simulink model "TST_EISGov_SelectTrqLim"  (R2016b)
settings: Solver=FixedStepDiscrete  StartTime=0.0  StopTime=simTime  FixedStep=sampleTime  RelTol=1e-3
values from neighbouring files (symbols this model uses):
  testCase = 1    [initTST_EISGov_SelectTrqLim_001.m]    (also in initTST_EISGov_SelectTrqLim_002.m = 2; initTST_EISGov_SelectTrqLim_003.m = 3)
libraries: simulink x19, UnitTest_Lib x15
settings Model: Creator=zhengjinyan  LastModifiedBy=zhengjinyan
settings DebuggingCC: SignalRangeChecking=error

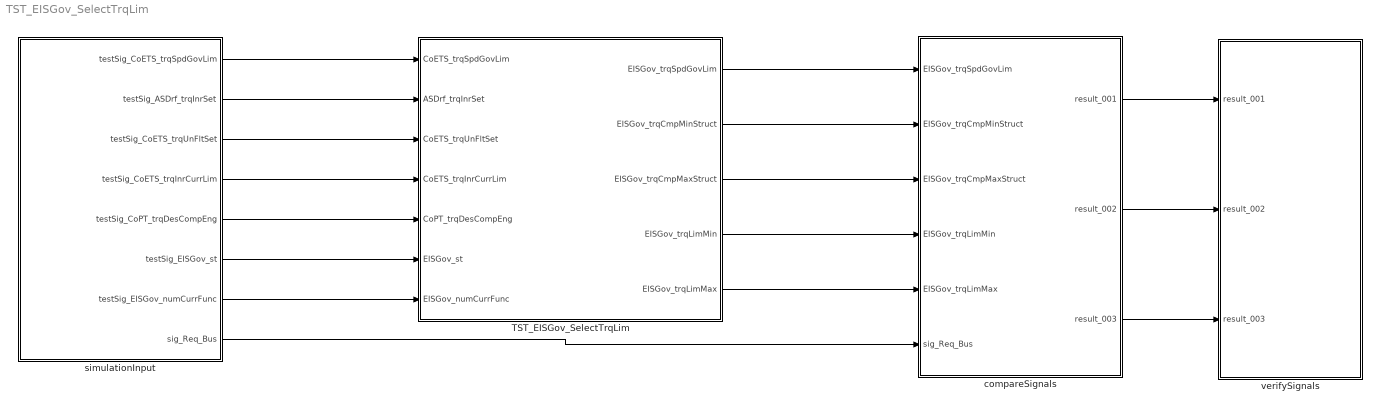
== system TST_EISGov_SelectTrqLim ==
  TST_EISGov_SelectTrqLim : Subsystem
  compareSignals : Subsystem
  simulationInput : Subsystem
  verifySignals : Subsystem
  wires:
  simulationInput/1(testSig_CoETS_trqSpdGovLim) -> TST_EISGov_SelectTrqLim/1(CoETS_trqSpdGovLim)
  simulationInput/2(testSig_ASDrf_trqInrSet) -> TST_EISGov_SelectTrqLim/2(ASDrf_trqInrSet)
  simulationInput/3(testSig_CoETS_trqUnFltSet) -> TST_EISGov_SelectTrqLim/3(CoETS_trqUnFltSet)
  simulationInput/4(testSig_CoETS_trqInrCurrLim) -> TST_EISGov_SelectTrqLim/4(CoETS_trqInrCurrLim)
  simulationInput/5(testSig_CoPT_trqDesCompEng) -> TST_EISGov_SelectTrqLim/5(CoPT_trqDesCompEng)
  simulationInput/6(testSig_EISGov_st) -> TST_EISGov_SelectTrqLim/6(EISGov_st)
  simulationInput/7(testSig_EISGov_numCurrFunc) -> TST_EISGov_SelectTrqLim/7(EISGov_numCurrFunc)
  TST_EISGov_SelectTrqLim/1(EISGov_trqSpdGovLim) -> compareSignals/1(EISGov_trqSpdGovLim)
  TST_EISGov_SelectTrqLim/2(EISGov_trqCmpMinStruct) -> compareSignals/2(EISGov_trqCmpMinStruct)
  TST_EISGov_SelectTrqLim/3(EISGov_trqCmpMaxStruct) -> compareSignals/3(EISGov_trqCmpMaxStruct)
  TST_EISGov_SelectTrqLim/4(EISGov_trqLimMin) -> compareSignals/4(EISGov_trqLimMin)
  TST_EISGov_SelectTrqLim/5(EISGov_trqLimMax) -> compareSignals/5(EISGov_trqLimMax)
  simulationInput/8(sig_Req_Bus) -> compareSignals/6(sig_Req_Bus)
  compareSignals/1(result_001) -> verifySignals/1(result_001)
  compareSignals/2(result_002) -> verifySignals/2(result_002)
  compareSignals/3(result_003) -> verifySignals/3(result_003)

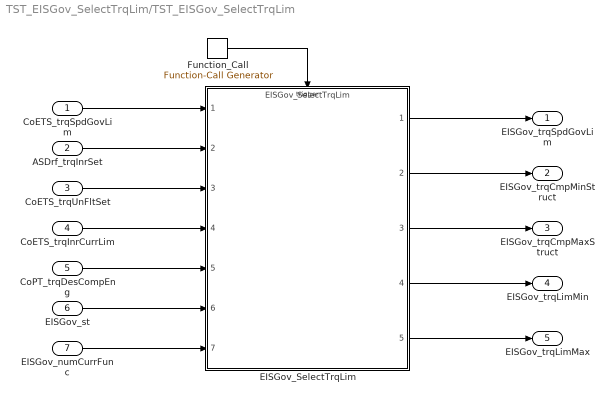
== system TST_EISGov_SelectTrqLim/TST_EISGov_SelectTrqLim ==
  CoETS_trqSpdGovLim : Inport
  ASDrf_trqInrSet : Inport  Port=2
  CoETS_trqUnFltSet : Inport  Port=3
  CoETS_trqInrCurrLim : Inport  Port=4
  CoPT_trqDesCompEng : Inport  Port=5
  EISGov_st : Inport  Port=6
  EISGov_numCurrFunc : Inport  Port=7
  EISGov_SelectTrqLim : ModelReference  ModelNameDialog=EISGov_SelectTrqLim  SimulationMode=Normal  ModelReferenceVersion=1.26  TriggerPortName=function  TriggerPortTriggerType=function-call  TriggerPortStatesWhenEnabling=held
  Function_Call : simulink/Ports & Subsystems/Function-Call Generator  sample_time=sampleTime  numberOfIterations=1
  EISGov_trqSpdGovLim : Outport
  EISGov_trqCmpMinStruct : Outport  Port=2
  EISGov_trqCmpMaxStruct : Outport  Port=3
  EISGov_trqLimMin : Outport  Port=4
  EISGov_trqLimMax : Outport  Port=5
  wires:
  Function_Call/1 -> EISGov_SelectTrqLim/Trigger
  CoETS_trqSpdGovLim/1 -> EISGov_SelectTrqLim/1
  ASDrf_trqInrSet/1 -> EISGov_SelectTrqLim/2
  CoETS_trqUnFltSet/1 -> EISGov_SelectTrqLim/3
  CoETS_trqInrCurrLim/1 -> EISGov_SelectTrqLim/4
  CoPT_trqDesCompEng/1 -> EISGov_SelectTrqLim/5
  EISGov_st/1 -> EISGov_SelectTrqLim/6
  EISGov_numCurrFunc/1 -> EISGov_SelectTrqLim/7
  EISGov_SelectTrqLim/1 -> EISGov_trqSpdGovLim/1
  EISGov_SelectTrqLim/2 -> EISGov_trqCmpMinStruct/1
  EISGov_SelectTrqLim/3 -> EISGov_trqCmpMaxStruct/1
  EISGov_SelectTrqLim/4 -> EISGov_trqLimMin/1
  EISGov_SelectTrqLim/5 -> EISGov_trqLimMax/1

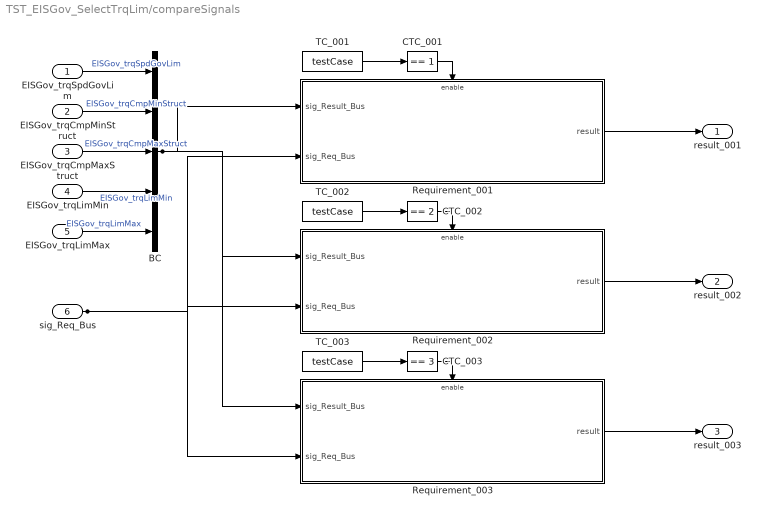
== system TST_EISGov_SelectTrqLim/compareSignals ==
  EISGov_trqSpdGovLim : Inport
  EISGov_trqCmpMinStruct : Inport  Port=2
  EISGov_trqCmpMaxStruct : Inport  Port=3
  EISGov_trqLimMin : Inport  Port=4
  EISGov_trqLimMax : Inport  Port=5
  sig_Req_Bus : Inport  Port=6
  BC : BusCreator  Inputs=5
  CTC_001 : simulink/Logic and Bit Operations/Compare To Constant  relop===  const=1  OutDataTypeStr=boolean
  CTC_002 : simulink/Logic and Bit Operations/Compare To Constant  relop===  const=2  OutDataTypeStr=boolean
  CTC_003 : simulink/Logic and Bit Operations/Compare To Constant  relop===  const=3  OutDataTypeStr=boolean
  Requirement_001 : Subsystem
  Requirement_002 : Subsystem
  Requirement_003 : Subsystem
  TC_001 : Constant  Value=testCase
  TC_002 : Constant  Value=testCase
  TC_003 : Constant  Value=testCase
  result_001 : Outport
  result_002 : Outport  Port=2
  result_003 : Outport  Port=3
  wires:
  EISGov_trqSpdGovLim/1 -> BC/1  "EISGov_trqSpdGovLim"
  EISGov_trqCmpMinStruct/1 -> BC/2  "EISGov_trqCmpMinStruct"
  EISGov_trqCmpMaxStruct/1 -> BC/3  "EISGov_trqCmpMaxStruct"
  EISGov_trqLimMin/1 -> BC/4  "EISGov_trqLimMin"
  EISGov_trqLimMax/1 -> BC/5  "EISGov_trqLimMax"
  TC_001/1 -> CTC_001/1
  CTC_001/1 -> Requirement_001/Enable
  sig_Req_Bus/1 -> Requirement_001/2(sig_Req_Bus), Requirement_002/2(sig_Req_Bus), Requirement_003/2(sig_Req_Bus)
  BC/1 -> Requirement_001/1(sig_Result_Bus), Requirement_002/1(sig_Result_Bus), Requirement_003/1(sig_Result_Bus)
  Requirement_001/1(result) -> result_001/1
  TC_002/1 -> CTC_002/1
  CTC_002/1 -> Requirement_002/Enable
  Requirement_002/1(result) -> result_002/1
  TC_003/1 -> CTC_003/1
  CTC_003/1 -> Requirement_003/Enable
  Requirement_003/1(result) -> result_003/1

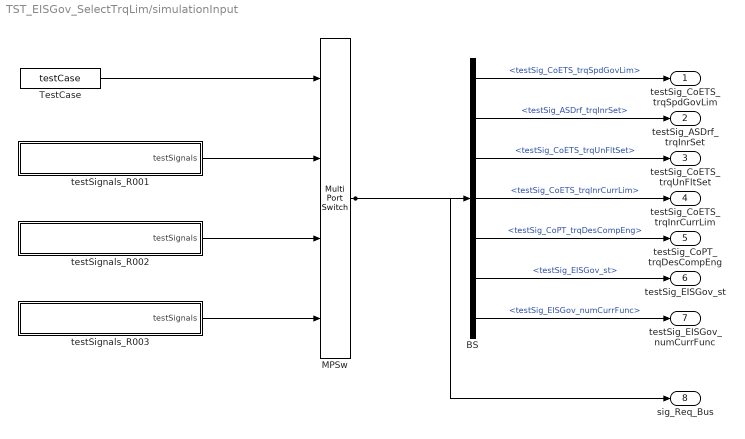
== system TST_EISGov_SelectTrqLim/simulationInput ==
  BS : BusSelector  OutputSignals=testSig_CoETS_trqSpdGovLim,testSig_ASDrf_trqInrSet,testSig_CoETS_trqUnFltSet,testSig_CoETS_trqInrCurrLim,testSig_CoPT_trqDesCompEng,testSig_EISGov_st,testSig_EISGov_numCurrFunc
  MPSw : MultiPortSwitch  SaturateOnIntegerOverflow=on  InputSameDT=on
  TestCase : Constant  Value=testCase
  testSignals_R001 : Subsystem
  testSignals_R002 : Subsystem
  testSignals_R003 : Subsystem
  testSig_CoETS_trqSpdGovLim : Outport
  testSig_ASDrf_trqInrSet : Outport  Port=2
  testSig_CoETS_trqUnFltSet : Outport  Port=3
  testSig_CoETS_trqInrCurrLim : Outport  Port=4
  testSig_CoPT_trqDesCompEng : Outport  Port=5
  testSig_EISGov_st : Outport  Port=6
  testSig_EISGov_numCurrFunc : Outport  Port=7
  sig_Req_Bus : Outport  Port=8
  wires:
  BS/1 -> testSig_CoETS_trqSpdGovLim/1  "<testSig_CoETS_trqSpdGovLim>"
  BS/2 -> testSig_ASDrf_trqInrSet/1  "<testSig_ASDrf_trqInrSet>"
  BS/3 -> testSig_CoETS_trqUnFltSet/1  "<testSig_CoETS_trqUnFltSet>"
  BS/4 -> testSig_CoETS_trqInrCurrLim/1  "<testSig_CoETS_trqInrCurrLim>"
  BS/5 -> testSig_CoPT_trqDesCompEng/1  "<testSig_CoPT_trqDesCompEng>"
  BS/6 -> testSig_EISGov_st/1  "<testSig_EISGov_st>"
  BS/7 -> testSig_EISGov_numCurrFunc/1  "<testSig_EISGov_numCurrFunc>"
  MPSw/1 -> BS/1, sig_Req_Bus/1
  TestCase/1 -> MPSw/1
  testSignals_R001/1(testSignals) -> MPSw/2
  testSignals_R002/1(testSignals) -> MPSw/3
  testSignals_R003/1(testSignals) -> MPSw/4

== system TST_EISGov_SelectTrqLim/verifySignals ==
  result_001 : Inport
  result_002 : Inport  Port=2
  result_003 : Inport  Port=3
  Assertion_001 : Assertion  Enabled=off
  Assertion_002 : Assertion  Enabled=off
  Assertion_003 : Assertion  Enabled=off
  wires:
  result_001/1 -> Assertion_001/1
  result_002/1 -> Assertion_002/1
  result_003/1 -> Assertion_003/1

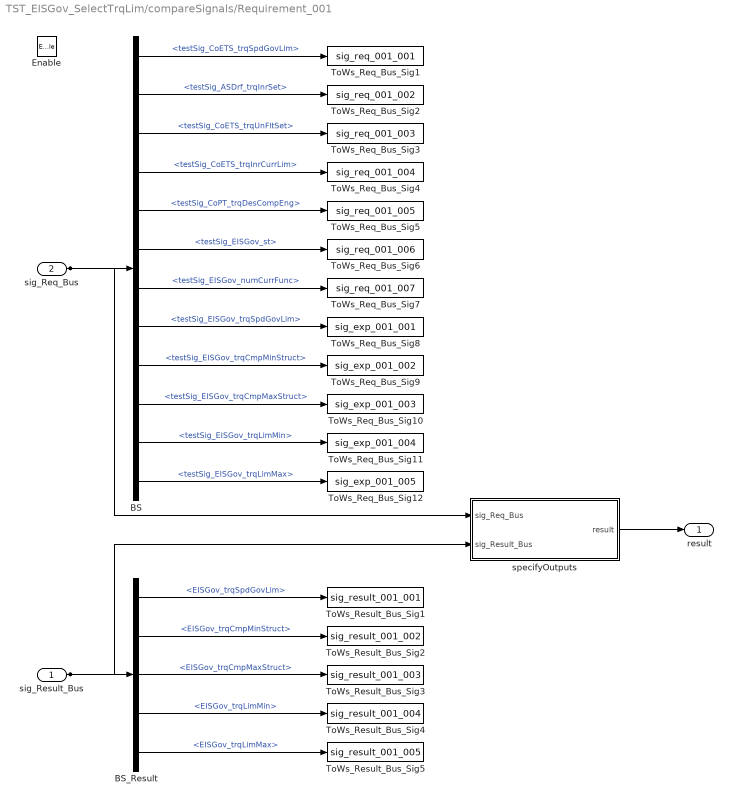
== system TST_EISGov_SelectTrqLim/compareSignals/Requirement_001 ==
  sig_Result_Bus : Inport
  sig_Req_Bus : Inport  Port=2
  Enable : EnablePort
  BS : BusSelector  OutputSignals=testSig_CoETS_trqSpdGovLim,testSig_ASDrf_trqInrSet,testSig_CoETS_trqUnFltSet,testSig_CoETS_trqInrCurrLim,testSig_CoPT_trqDesCompEng,testSig_EISGov_st,testSig_EISGov_numCurrFunc,testSig_EISGov_trqSpdGovLim,testSig_EISGov_trqCmpMinStruct,testSig_EISGov_trqCmpMaxStruct,testSig_EISGov_trqLimMin,testSig_EISGov_trqLimMax
  BS_Result : BusSelector  OutputSignals=EISGov_trqSpdGovLim,EISGov_trqCmpMinStruct,EISGov_trqCmpMaxStruct,EISGov_trqLimMin,EISGov_trqLimMax
  ToWs_Req_Bus_Sig1 : ToWorkspace  VariableName=sig_req_001_001  SaveFormat=Structure With Time
  ToWs_Req_Bus_Sig10 : ToWorkspace  VariableName=sig_exp_001_003  SaveFormat=Structure With Time
  ToWs_Req_Bus_Sig11 : ToWorkspace  VariableName=sig_exp_001_004  SaveFormat=Structure With Time
  ToWs_Req_Bus_Sig12 : ToWorkspace  VariableName=sig_exp_001_005  SaveFormat=Structure With Time
  ToWs_Req_Bus_Sig2 : ToWorkspace  VariableName=sig_req_001_002  SaveFormat=Structure With Time
  ToWs_Req_Bus_Sig3 : ToWorkspace  VariableName=sig_req_001_003  SaveFormat=Structure With Time
  ToWs_Req_Bus_Sig4 : ToWorkspace  VariableName=sig_req_001_004  SaveFormat=Structure With Time
  ToWs_Req_Bus_Sig5 : ToWorkspace  VariableName=sig_req_001_005  SaveFormat=Structure With Time
  ToWs_Req_Bus_Sig6 : ToWorkspace  VariableName=sig_req_001_006  SaveFormat=Structure With Time
  ToWs_Req_Bus_Sig7 : ToWorkspace  VariableName=sig_req_001_007  SaveFormat=Structure With Time
  ToWs_Req_Bus_Sig8 : ToWorkspace  VariableName=sig_exp_001_001  SaveFormat=Structure With Time
  ToWs_Req_Bus_Sig9 : ToWorkspace  VariableName=sig_exp_001_002  SaveFormat=Structure With Time
  ToWs_Result_Bus_Sig1 : ToWorkspace  VariableName=sig_result_001_001  SaveFormat=Structure With Time
  ToWs_Result_Bus_Sig2 : ToWorkspace  VariableName=sig_result_001_002  SaveFormat=Structure With Time
  ToWs_Result_Bus_Sig3 : ToWorkspace  VariableName=sig_result_001_003  SaveFormat=Structure With Time
  ToWs_Result_Bus_Sig4 : ToWorkspace  VariableName=sig_result_001_004  SaveFormat=Structure With Time
  ToWs_Result_Bus_Sig5 : ToWorkspace  VariableName=sig_result_001_005  SaveFormat=Structure With Time
  specifyOutputs : Subsystem
  result : Outport
  wires:
  sig_Req_Bus/1 -> BS/1, specifyOutputs/1(sig_Req_Bus)
  BS/1 -> ToWs_Req_Bus_Sig1/1  "<testSig_CoETS_trqSpdGovLim>"
  BS/2 -> ToWs_Req_Bus_Sig2/1  "<testSig_ASDrf_trqInrSet>"
  BS/3 -> ToWs_Req_Bus_Sig3/1  "<testSig_CoETS_trqUnFltSet>"
  BS/4 -> ToWs_Req_Bus_Sig4/1  "<testSig_CoETS_trqInrCurrLim>"
  BS/5 -> ToWs_Req_Bus_Sig5/1  "<testSig_CoPT_trqDesCompEng>"
  BS/6 -> ToWs_Req_Bus_Sig6/1  "<testSig_EISGov_st>"
  BS/7 -> ToWs_Req_Bus_Sig7/1  "<testSig_EISGov_numCurrFunc>"
  BS/8 -> ToWs_Req_Bus_Sig8/1  "<testSig_EISGov_trqSpdGovLim>"
  BS/9 -> ToWs_Req_Bus_Sig9/1  "<testSig_EISGov_trqCmpMinStruct>"
  BS/10 -> ToWs_Req_Bus_Sig10/1  "<testSig_EISGov_trqCmpMaxStruct>"
  BS/11 -> ToWs_Req_Bus_Sig11/1  "<testSig_EISGov_trqLimMin>"
  BS/12 -> ToWs_Req_Bus_Sig12/1  "<testSig_EISGov_trqLimMax>"
  sig_Result_Bus/1 -> BS_Result/1, specifyOutputs/2(sig_Result_Bus)
  BS_Result/1 -> ToWs_Result_Bus_Sig1/1  "<EISGov_trqSpdGovLim>"
  BS_Result/2 -> ToWs_Result_Bus_Sig2/1  "<EISGov_trqCmpMinStruct>"
  BS_Result/3 -> ToWs_Result_Bus_Sig3/1  "<EISGov_trqCmpMaxStruct>"
  BS_Result/4 -> ToWs_Result_Bus_Sig4/1  "<EISGov_trqLimMin>"
  BS_Result/5 -> ToWs_Result_Bus_Sig5/1  "<EISGov_trqLimMax>"
  specifyOutputs/1(result) -> result/1

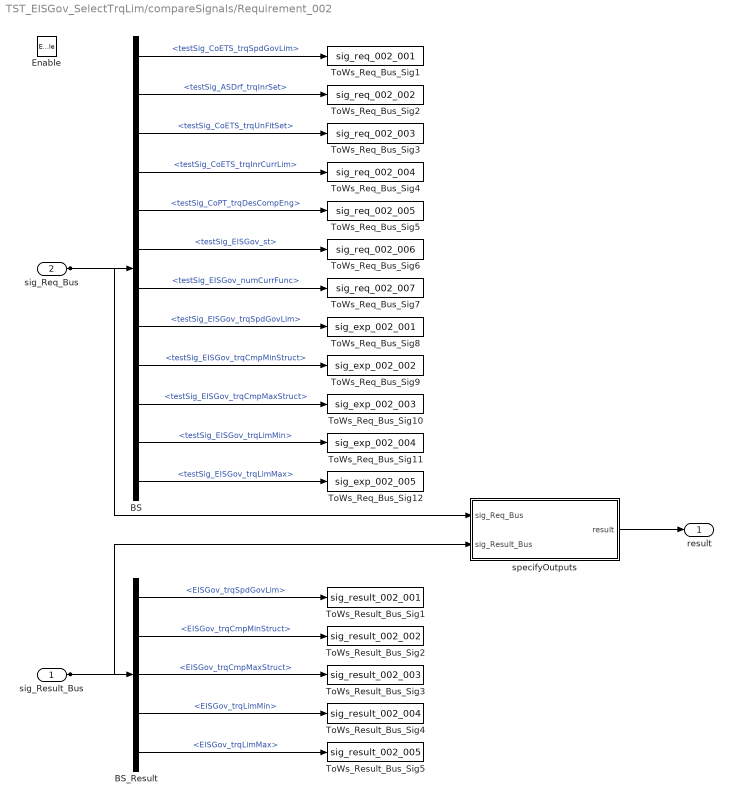
== system TST_EISGov_SelectTrqLim/compareSignals/Requirement_002 ==
  sig_Result_Bus : Inport
  sig_Req_Bus : Inport  Port=2
  Enable : EnablePort
  BS : BusSelector  OutputSignals=testSig_CoETS_trqSpdGovLim,testSig_ASDrf_trqInrSet,testSig_CoETS_trqUnFltSet,testSig_CoETS_trqInrCurrLim,testSig_CoPT_trqDesCompEng,testSig_EISGov_st,testSig_EISGov_numCurrFunc,testSig_EISGov_trqSpdGovLim,testSig_EISGov_trqCmpMinStruct,testSig_EISGov_trqCmpMaxStruct,testSig_EISGov_trqLimMin,testSig_EISGov_trqLimMax
  BS_Result : BusSelector  OutputSignals=EISGov_trqSpdGovLim,EISGov_trqCmpMinStruct,EISGov_trqCmpMaxStruct,EISGov_trqLimMin,EISGov_trqLimMax
  ToWs_Req_Bus_Sig1 : ToWorkspace  VariableName=sig_req_002_001  SaveFormat=Structure With Time
  ToWs_Req_Bus_Sig10 : ToWorkspace  VariableName=sig_exp_002_003  SaveFormat=Structure With Time
  ToWs_Req_Bus_Sig11 : ToWorkspace  VariableName=sig_exp_002_004  SaveFormat=Structure With Time
  ToWs_Req_Bus_Sig12 : ToWorkspace  VariableName=sig_exp_002_005  SaveFormat=Structure With Time
  ToWs_Req_Bus_Sig2 : ToWorkspace  VariableName=sig_req_002_002  SaveFormat=Structure With Time
  ToWs_Req_Bus_Sig3 : ToWorkspace  VariableName=sig_req_002_003  SaveFormat=Structure With Time
  ToWs_Req_Bus_Sig4 : ToWorkspace  VariableName=sig_req_002_004  SaveFormat=Structure With Time
  ToWs_Req_Bus_Sig5 : ToWorkspace  VariableName=sig_req_002_005  SaveFormat=Structure With Time
  ToWs_Req_Bus_Sig6 : ToWorkspace  VariableName=sig_req_002_006  SaveFormat=Structure With Time
  ToWs_Req_Bus_Sig7 : ToWorkspace  VariableName=sig_req_002_007  SaveFormat=Structure With Time
  ToWs_Req_Bus_Sig8 : ToWorkspace  VariableName=sig_exp_002_001  SaveFormat=Structure With Time
  ToWs_Req_Bus_Sig9 : ToWorkspace  VariableName=sig_exp_002_002  SaveFormat=Structure With Time
  ToWs_Result_Bus_Sig1 : ToWorkspace  VariableName=sig_result_002_001  SaveFormat=Structure With Time
  ToWs_Result_Bus_Sig2 : ToWorkspace  VariableName=sig_result_002_002  SaveFormat=Structure With Time
  ToWs_Result_Bus_Sig3 : ToWorkspace  VariableName=sig_result_002_003  SaveFormat=Structure With Time
  ToWs_Result_Bus_Sig4 : ToWorkspace  VariableName=sig_result_002_004  SaveFormat=Structure With Time
  ToWs_Result_Bus_Sig5 : ToWorkspace  VariableName=sig_result_002_005  SaveFormat=Structure With Time
  specifyOutputs : Subsystem
  result : Outport
  wires:
  sig_Req_Bus/1 -> BS/1, specifyOutputs/1(sig_Req_Bus)
  BS/1 -> ToWs_Req_Bus_Sig1/1  "<testSig_CoETS_trqSpdGovLim>"
  BS/2 -> ToWs_Req_Bus_Sig2/1  "<testSig_ASDrf_trqInrSet>"
  BS/3 -> ToWs_Req_Bus_Sig3/1  "<testSig_CoETS_trqUnFltSet>"
  BS/4 -> ToWs_Req_Bus_Sig4/1  "<testSig_CoETS_trqInrCurrLim>"
  BS/5 -> ToWs_Req_Bus_Sig5/1  "<testSig_CoPT_trqDesCompEng>"
  BS/6 -> ToWs_Req_Bus_Sig6/1  "<testSig_EISGov_st>"
  BS/7 -> ToWs_Req_Bus_Sig7/1  "<testSig_EISGov_numCurrFunc>"
  BS/8 -> ToWs_Req_Bus_Sig8/1  "<testSig_EISGov_trqSpdGovLim>"
  BS/9 -> ToWs_Req_Bus_Sig9/1  "<testSig_EISGov_trqCmpMinStruct>"
  BS/10 -> ToWs_Req_Bus_Sig10/1  "<testSig_EISGov_trqCmpMaxStruct>"
  BS/11 -> ToWs_Req_Bus_Sig11/1  "<testSig_EISGov_trqLimMin>"
  BS/12 -> ToWs_Req_Bus_Sig12/1  "<testSig_EISGov_trqLimMax>"
  sig_Result_Bus/1 -> BS_Result/1, specifyOutputs/2(sig_Result_Bus)
  BS_Result/1 -> ToWs_Result_Bus_Sig1/1  "<EISGov_trqSpdGovLim>"
  BS_Result/2 -> ToWs_Result_Bus_Sig2/1  "<EISGov_trqCmpMinStruct>"
  BS_Result/3 -> ToWs_Result_Bus_Sig3/1  "<EISGov_trqCmpMaxStruct>"
  BS_Result/4 -> ToWs_Result_Bus_Sig4/1  "<EISGov_trqLimMin>"
  BS_Result/5 -> ToWs_Result_Bus_Sig5/1  "<EISGov_trqLimMax>"
  specifyOutputs/1(result) -> result/1

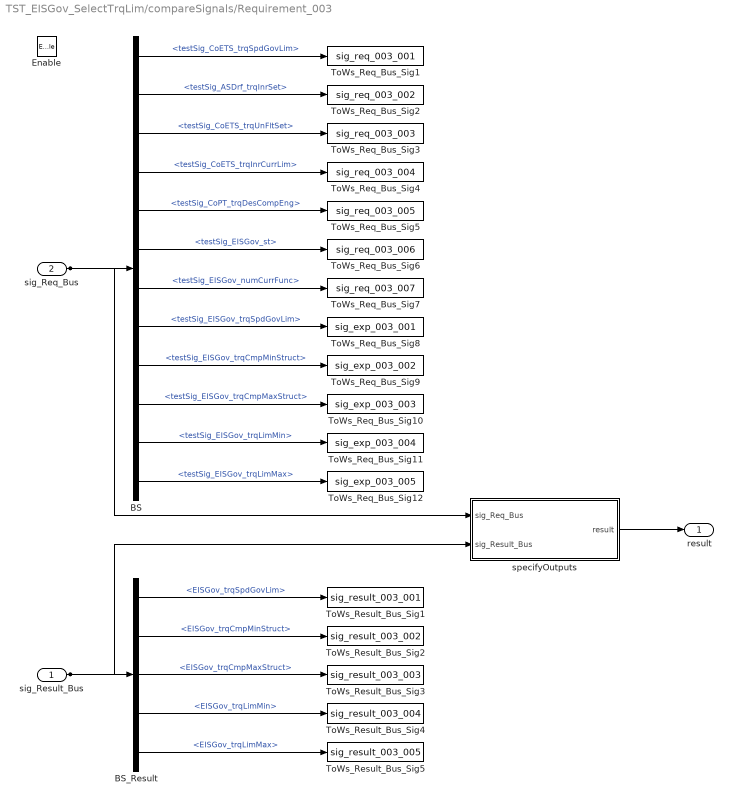
== system TST_EISGov_SelectTrqLim/compareSignals/Requirement_003 ==
  sig_Result_Bus : Inport
  sig_Req_Bus : Inport  Port=2
  Enable : EnablePort
  BS : BusSelector  OutputSignals=testSig_CoETS_trqSpdGovLim,testSig_ASDrf_trqInrSet,testSig_CoETS_trqUnFltSet,testSig_CoETS_trqInrCurrLim,testSig_CoPT_trqDesCompEng,testSig_EISGov_st,testSig_EISGov_numCurrFunc,testSig_EISGov_trqSpdGovLim,testSig_EISGov_trqCmpMinStruct,testSig_EISGov_trqCmpMaxStruct,testSig_EISGov_trqLimMin,testSig_EISGov_trqLimMax
  BS_Result : BusSelector  OutputSignals=EISGov_trqSpdGovLim,EISGov_trqCmpMinStruct,EISGov_trqCmpMaxStruct,EISGov_trqLimMin,EISGov_trqLimMax
  ToWs_Req_Bus_Sig1 : ToWorkspace  VariableName=sig_req_003_001  SaveFormat=Structure With Time
  ToWs_Req_Bus_Sig10 : ToWorkspace  VariableName=sig_exp_003_003  SaveFormat=Structure With Time
  ToWs_Req_Bus_Sig11 : ToWorkspace  VariableName=sig_exp_003_004  SaveFormat=Structure With Time
  ToWs_Req_Bus_Sig12 : ToWorkspace  VariableName=sig_exp_003_005  SaveFormat=Structure With Time
  ToWs_Req_Bus_Sig2 : ToWorkspace  VariableName=sig_req_003_002  SaveFormat=Structure With Time
  ToWs_Req_Bus_Sig3 : ToWorkspace  VariableName=sig_req_003_003  SaveFormat=Structure With Time
  ToWs_Req_Bus_Sig4 : ToWorkspace  VariableName=sig_req_003_004  SaveFormat=Structure With Time
  ToWs_Req_Bus_Sig5 : ToWorkspace  VariableName=sig_req_003_005  SaveFormat=Structure With Time
  ToWs_Req_Bus_Sig6 : ToWorkspace  VariableName=sig_req_003_006  SaveFormat=Structure With Time
  ToWs_Req_Bus_Sig7 : ToWorkspace  VariableName=sig_req_003_007  SaveFormat=Structure With Time
  ToWs_Req_Bus_Sig8 : ToWorkspace  VariableName=sig_exp_003_001  SaveFormat=Structure With Time
  ToWs_Req_Bus_Sig9 : ToWorkspace  VariableName=sig_exp_003_002  SaveFormat=Structure With Time
  ToWs_Result_Bus_Sig1 : ToWorkspace  VariableName=sig_result_003_001  SaveFormat=Structure With Time
  ToWs_Result_Bus_Sig2 : ToWorkspace  VariableName=sig_result_003_002  SaveFormat=Structure With Time
  ToWs_Result_Bus_Sig3 : ToWorkspace  VariableName=sig_result_003_003  SaveFormat=Structure With Time
  ToWs_Result_Bus_Sig4 : ToWorkspace  VariableName=sig_result_003_004  SaveFormat=Structure With Time
  ToWs_Result_Bus_Sig5 : ToWorkspace  VariableName=sig_result_003_005  SaveFormat=Structure With Time
  specifyOutputs : Subsystem
  result : Outport
  wires:
  sig_Req_Bus/1 -> BS/1, specifyOutputs/1(sig_Req_Bus)
  BS/1 -> ToWs_Req_Bus_Sig1/1  "<testSig_CoETS_trqSpdGovLim>"
  BS/2 -> ToWs_Req_Bus_Sig2/1  "<testSig_ASDrf_trqInrSet>"
  BS/3 -> ToWs_Req_Bus_Sig3/1  "<testSig_CoETS_trqUnFltSet>"
  BS/4 -> ToWs_Req_Bus_Sig4/1  "<testSig_CoETS_trqInrCurrLim>"
  BS/5 -> ToWs_Req_Bus_Sig5/1  "<testSig_CoPT_trqDesCompEng>"
  BS/6 -> ToWs_Req_Bus_Sig6/1  "<testSig_EISGov_st>"
  BS/7 -> ToWs_Req_Bus_Sig7/1  "<testSig_EISGov_numCurrFunc>"
  BS/8 -> ToWs_Req_Bus_Sig8/1  "<testSig_EISGov_trqSpdGovLim>"
  BS/9 -> ToWs_Req_Bus_Sig9/1  "<testSig_EISGov_trqCmpMinStruct>"
  BS/10 -> ToWs_Req_Bus_Sig10/1  "<testSig_EISGov_trqCmpMaxStruct>"
  BS/11 -> ToWs_Req_Bus_Sig11/1  "<testSig_EISGov_trqLimMin>"
  BS/12 -> ToWs_Req_Bus_Sig12/1  "<testSig_EISGov_trqLimMax>"
  sig_Result_Bus/1 -> BS_Result/1, specifyOutputs/2(sig_Result_Bus)
  BS_Result/1 -> ToWs_Result_Bus_Sig1/1  "<EISGov_trqSpdGovLim>"
  BS_Result/2 -> ToWs_Result_Bus_Sig2/1  "<EISGov_trqCmpMinStruct>"
  BS_Result/3 -> ToWs_Result_Bus_Sig3/1  "<EISGov_trqCmpMaxStruct>"
  BS_Result/4 -> ToWs_Result_Bus_Sig4/1  "<EISGov_trqLimMin>"
  BS_Result/5 -> ToWs_Result_Bus_Sig5/1  "<EISGov_trqLimMax>"
  specifyOutputs/1(result) -> result/1

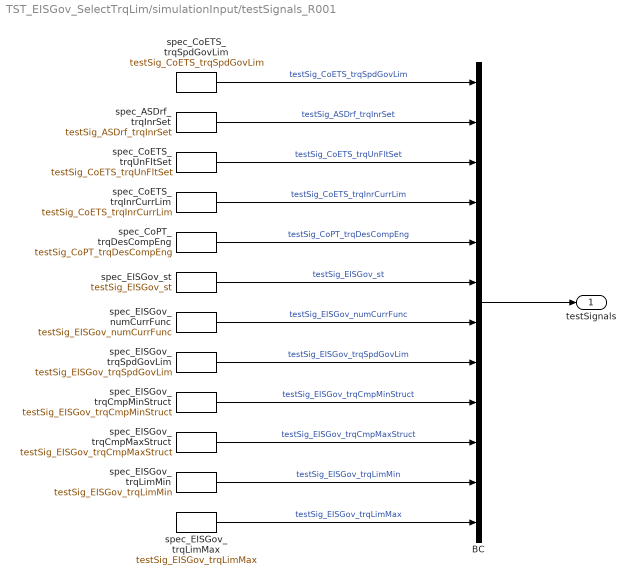
== system TST_EISGov_SelectTrqLim/simulationInput/testSignals_R001 ==
  BC : BusCreator  Inputs=12
  spec_ASDrf_trqInrSet : FromWorkspace  VariableName=testSig_ASDrf_trqInrSet  Interpolate=off  OutputAfterFinalValue=Holding final value
  spec_CoETS_trqInrCurrLim : FromWorkspace  VariableName=testSig_CoETS_trqInrCurrLim  Interpolate=off  OutputAfterFinalValue=Holding final value
  spec_CoETS_trqSpdGovLim : FromWorkspace  VariableName=testSig_CoETS_trqSpdGovLim  Interpolate=off  OutputAfterFinalValue=Holding final value
  spec_CoETS_trqUnFltSet : FromWorkspace  VariableName=testSig_CoETS_trqUnFltSet  Interpolate=off  OutputAfterFinalValue=Holding final value
  spec_CoPT_trqDesCompEng : FromWorkspace  VariableName=testSig_CoPT_trqDesCompEng  Interpolate=off  OutputAfterFinalValue=Holding final value
  spec_EISGov_numCurrFunc : FromWorkspace  VariableName=testSig_EISGov_numCurrFunc  Interpolate=off  OutputAfterFinalValue=Holding final value
  spec_EISGov_st : FromWorkspace  VariableName=testSig_EISGov_st  Interpolate=off  OutputAfterFinalValue=Holding final value
  spec_EISGov_trqCmpMaxStruct : FromWorkspace  VariableName=testSig_EISGov_trqCmpMaxStruct  Interpolate=off  OutputAfterFinalValue=Holding final value
  spec_EISGov_trqCmpMinStruct : FromWorkspace  VariableName=testSig_EISGov_trqCmpMinStruct  Interpolate=off  OutputAfterFinalValue=Holding final value
  spec_EISGov_trqLimMax : FromWorkspace  VariableName=testSig_EISGov_trqLimMax  Interpolate=off  OutputAfterFinalValue=Holding final value
  spec_EISGov_trqLimMin : FromWorkspace  VariableName=testSig_EISGov_trqLimMin  Interpolate=off  OutputAfterFinalValue=Holding final value
  spec_EISGov_trqSpdGovLim : FromWorkspace  VariableName=testSig_EISGov_trqSpdGovLim  Interpolate=off  OutputAfterFinalValue=Holding final value
  testSignals : Outport
  wires:
  BC/1 -> testSignals/1
  spec_CoETS_trqSpdGovLim/1 -> BC/1  "testSig_CoETS_trqSpdGovLim"
  spec_ASDrf_trqInrSet/1 -> BC/2  "testSig_ASDrf_trqInrSet"
  spec_CoETS_trqUnFltSet/1 -> BC/3  "testSig_CoETS_trqUnFltSet"
  spec_CoETS_trqInrCurrLim/1 -> BC/4  "testSig_CoETS_trqInrCurrLim"
  spec_CoPT_trqDesCompEng/1 -> BC/5  "testSig_CoPT_trqDesCompEng"
  spec_EISGov_st/1 -> BC/6  "testSig_EISGov_st"
  spec_EISGov_numCurrFunc/1 -> BC/7  "testSig_EISGov_numCurrFunc"
  spec_EISGov_trqSpdGovLim/1 -> BC/8  "testSig_EISGov_trqSpdGovLim"
  spec_EISGov_trqCmpMinStruct/1 -> BC/9  "testSig_EISGov_trqCmpMinStruct"
  spec_EISGov_trqCmpMaxStruct/1 -> BC/10  "testSig_EISGov_trqCmpMaxStruct"
  spec_EISGov_trqLimMin/1 -> BC/11  "testSig_EISGov_trqLimMin"
  spec_EISGov_trqLimMax/1 -> BC/12  "testSig_EISGov_trqLimMax"

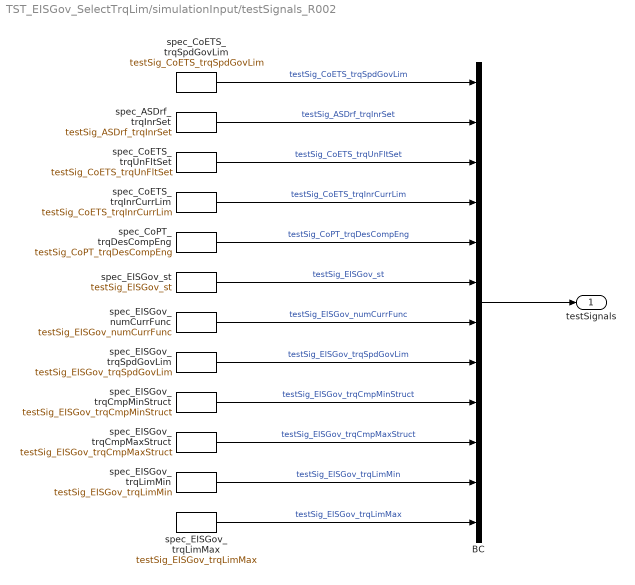
== system TST_EISGov_SelectTrqLim/simulationInput/testSignals_R002 ==
  BC : BusCreator  Inputs=12
  spec_ASDrf_trqInrSet : FromWorkspace  VariableName=testSig_ASDrf_trqInrSet  Interpolate=off  OutputAfterFinalValue=Holding final value
  spec_CoETS_trqInrCurrLim : FromWorkspace  VariableName=testSig_CoETS_trqInrCurrLim  Interpolate=off  OutputAfterFinalValue=Holding final value
  spec_CoETS_trqSpdGovLim : FromWorkspace  VariableName=testSig_CoETS_trqSpdGovLim  Interpolate=off  OutputAfterFinalValue=Holding final value
  spec_CoETS_trqUnFltSet : FromWorkspace  VariableName=testSig_CoETS_trqUnFltSet  Interpolate=off  OutputAfterFinalValue=Holding final value
  spec_CoPT_trqDesCompEng : FromWorkspace  VariableName=testSig_CoPT_trqDesCompEng  Interpolate=off  OutputAfterFinalValue=Holding final value
  spec_EISGov_numCurrFunc : FromWorkspace  VariableName=testSig_EISGov_numCurrFunc  Interpolate=off  OutputAfterFinalValue=Holding final value
  spec_EISGov_st : FromWorkspace  VariableName=testSig_EISGov_st  Interpolate=off  OutputAfterFinalValue=Holding final value
  spec_EISGov_trqCmpMaxStruct : FromWorkspace  VariableName=testSig_EISGov_trqCmpMaxStruct  Interpolate=off  OutputAfterFinalValue=Holding final value
  spec_EISGov_trqCmpMinStruct : FromWorkspace  VariableName=testSig_EISGov_trqCmpMinStruct  Interpolate=off  OutputAfterFinalValue=Holding final value
  spec_EISGov_trqLimMax : FromWorkspace  VariableName=testSig_EISGov_trqLimMax  Interpolate=off  OutputAfterFinalValue=Holding final value
  spec_EISGov_trqLimMin : FromWorkspace  VariableName=testSig_EISGov_trqLimMin  Interpolate=off  OutputAfterFinalValue=Holding final value
  spec_EISGov_trqSpdGovLim : FromWorkspace  VariableName=testSig_EISGov_trqSpdGovLim  Interpolate=off  OutputAfterFinalValue=Holding final value
  testSignals : Outport
  wires:
  BC/1 -> testSignals/1
  spec_CoETS_trqSpdGovLim/1 -> BC/1  "testSig_CoETS_trqSpdGovLim"
  spec_ASDrf_trqInrSet/1 -> BC/2  "testSig_ASDrf_trqInrSet"
  spec_CoETS_trqUnFltSet/1 -> BC/3  "testSig_CoETS_trqUnFltSet"
  spec_CoETS_trqInrCurrLim/1 -> BC/4  "testSig_CoETS_trqInrCurrLim"
  spec_CoPT_trqDesCompEng/1 -> BC/5  "testSig_CoPT_trqDesCompEng"
  spec_EISGov_st/1 -> BC/6  "testSig_EISGov_st"
  spec_EISGov_numCurrFunc/1 -> BC/7  "testSig_EISGov_numCurrFunc"
  spec_EISGov_trqSpdGovLim/1 -> BC/8  "testSig_EISGov_trqSpdGovLim"
  spec_EISGov_trqCmpMinStruct/1 -> BC/9  "testSig_EISGov_trqCmpMinStruct"
  spec_EISGov_trqCmpMaxStruct/1 -> BC/10  "testSig_EISGov_trqCmpMaxStruct"
  spec_EISGov_trqLimMin/1 -> BC/11  "testSig_EISGov_trqLimMin"
  spec_EISGov_trqLimMax/1 -> BC/12  "testSig_EISGov_trqLimMax"

== system TST_EISGov_SelectTrqLim/simulationInput/testSignals_R003 ==
  BC : BusCreator  Inputs=12
  spec_ASDrf_trqInrSet : FromWorkspace  VariableName=testSig_ASDrf_trqInrSet  Interpolate=off  OutputAfterFinalValue=Holding final value
  spec_CoETS_trqInrCurrLim : FromWorkspace  VariableName=testSig_CoETS_trqInrCurrLim  Interpolate=off  OutputAfterFinalValue=Holding final value
  spec_CoETS_trqSpdGovLim : FromWorkspace  VariableName=testSig_CoETS_trqSpdGovLim  Interpolate=off  OutputAfterFinalValue=Holding final value
  spec_CoETS_trqUnFltSet : FromWorkspace  VariableName=testSig_CoETS_trqUnFltSet  Interpolate=off  OutputAfterFinalValue=Holding final value
  spec_CoPT_trqDesCompEng : FromWorkspace  VariableName=testSig_CoPT_trqDesCompEng  Interpolate=off  OutputAfterFinalValue=Holding final value
  spec_EISGov_numCurrFunc : FromWorkspace  VariableName=testSig_EISGov_numCurrFunc  Interpolate=off  OutputAfterFinalValue=Holding final value
  spec_EISGov_st : FromWorkspace  VariableName=testSig_EISGov_st  Interpolate=off  OutputAfterFinalValue=Holding final value
  spec_EISGov_trqCmpMaxStruct : FromWorkspace  VariableName=testSig_EISGov_trqCmpMaxStruct  Interpolate=off  OutputAfterFinalValue=Holding final value
  spec_EISGov_trqCmpMinStruct : FromWorkspace  VariableName=testSig_EISGov_trqCmpMinStruct  Interpolate=off  OutputAfterFinalValue=Holding final value
  spec_EISGov_trqLimMax : FromWorkspace  VariableName=testSig_EISGov_trqLimMax  Interpolate=off  OutputAfterFinalValue=Holding final value
  spec_EISGov_trqLimMin : FromWorkspace  VariableName=testSig_EISGov_trqLimMin  Interpolate=off  OutputAfterFinalValue=Holding final value
  spec_EISGov_trqSpdGovLim : FromWorkspace  VariableName=testSig_EISGov_trqSpdGovLim  Interpolate=off  OutputAfterFinalValue=Holding final value
  testSignals : Outport
  wires:
  BC/1 -> testSignals/1
  spec_CoETS_trqSpdGovLim/1 -> BC/1  "testSig_CoETS_trqSpdGovLim"
  spec_ASDrf_trqInrSet/1 -> BC/2  "testSig_ASDrf_trqInrSet"
  spec_CoETS_trqUnFltSet/1 -> BC/3  "testSig_CoETS_trqUnFltSet"
  spec_CoETS_trqInrCurrLim/1 -> BC/4  "testSig_CoETS_trqInrCurrLim"
  spec_CoPT_trqDesCompEng/1 -> BC/5  "testSig_CoPT_trqDesCompEng"
  spec_EISGov_st/1 -> BC/6  "testSig_EISGov_st"
  spec_EISGov_numCurrFunc/1 -> BC/7  "testSig_EISGov_numCurrFunc"
  spec_EISGov_trqSpdGovLim/1 -> BC/8  "testSig_EISGov_trqSpdGovLim"
  spec_EISGov_trqCmpMinStruct/1 -> BC/9  "testSig_EISGov_trqCmpMinStruct"
  spec_EISGov_trqCmpMaxStruct/1 -> BC/10  "testSig_EISGov_trqCmpMaxStruct"
  spec_EISGov_trqLimMin/1 -> BC/11  "testSig_EISGov_trqLimMin"
  spec_EISGov_trqLimMax/1 -> BC/12  "testSig_EISGov_trqLimMax"

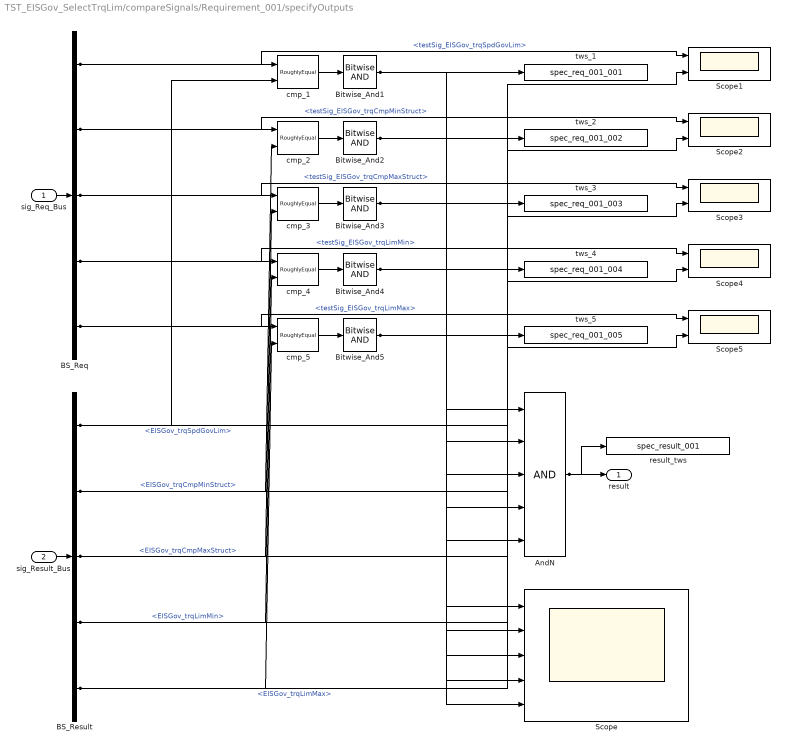
== system TST_EISGov_SelectTrqLim/compareSignals/Requirement_001/specifyOutputs ==
  sig_Req_Bus : Inport
  sig_Result_Bus : Inport  Port=2
  AndN : Logic  Inputs=5
  BS_Req : BusSelector  OutputSignals=testSig_EISGov_trqSpdGovLim,testSig_EISGov_trqCmpMinStruct,testSig_EISGov_trqCmpMaxStruct,testSig_EISGov_trqLimMin,testSig_EISGov_trqLimMax
  BS_Result : BusSelector  OutputSignals=EISGov_trqSpdGovLim,EISGov_trqCmpMinStruct,EISGov_trqCmpMaxStruct,EISGov_trqLimMin,EISGov_trqLimMax
  Bitwise_And{1..5} (5 alike) : simulink/Logic and Bit Operations/Bitwise Operator  logicop=AND  UseBitMask=off  BitMask=bin2dec('11011001')  BitMaskRealWorld=Stored Integer
  Scope : Scope  NumInputPorts=5
  Scope{1..5} (5 alike) : Scope  NumInputPorts=2
  cmp_{1..5} (5 alike) : UnitTest_Lib/RoughlyEqual  slope=0.1
  result_tws : ToWorkspace  VariableName=spec_result_001
  tws_1 : ToWorkspace  VariableName=spec_req_001_001
  tws_2 : ToWorkspace  VariableName=spec_req_001_002
  tws_3 : ToWorkspace  VariableName=spec_req_001_003
  tws_4 : ToWorkspace  VariableName=spec_req_001_004
  tws_5 : ToWorkspace  VariableName=spec_req_001_005
  result : Outport
  wires:
  sig_Req_Bus/1 -> BS_Req/1
  sig_Result_Bus/1 -> BS_Result/1
  AndN/1 -> result/1, result_tws/1
  BS_Req/1 -> cmp_1/1, Scope1/1  "<testSig_EISGov_trqSpdGovLim>"
  BS_Result/1 -> cmp_1/2, Scope1/2  "<EISGov_trqSpdGovLim>"
  cmp_1/1 -> Bitwise_And1/1
  Bitwise_And1/1 -> tws_1/1, AndN/1, Scope/1
  BS_Req/2 -> cmp_2/1, Scope2/1  "<testSig_EISGov_trqCmpMinStruct>"
  BS_Result/2 -> cmp_2/2, Scope2/2  "<EISGov_trqCmpMinStruct>"
  cmp_2/1 -> Bitwise_And2/1
  Bitwise_And2/1 -> tws_2/1, AndN/2, Scope/2
  BS_Req/3 -> cmp_3/1, Scope3/1  "<testSig_EISGov_trqCmpMaxStruct>"
  BS_Result/3 -> cmp_3/2, Scope3/2  "<EISGov_trqCmpMaxStruct>"
  cmp_3/1 -> Bitwise_And3/1
  Bitwise_And3/1 -> tws_3/1, AndN/3, Scope/3
  BS_Req/4 -> cmp_4/1, Scope4/1  "<testSig_EISGov_trqLimMin>"
  BS_Result/4 -> cmp_4/2, Scope4/2  "<EISGov_trqLimMin>"
  cmp_4/1 -> Bitwise_And4/1
  Bitwise_And4/1 -> tws_4/1, AndN/4, Scope/4
  BS_Req/5 -> cmp_5/1, Scope5/1  "<testSig_EISGov_trqLimMax>"
  BS_Result/5 -> cmp_5/2, Scope5/2  "<EISGov_trqLimMax>"
  cmp_5/1 -> Bitwise_And5/1
  Bitwise_And5/1 -> tws_5/1, AndN/5, Scope/5

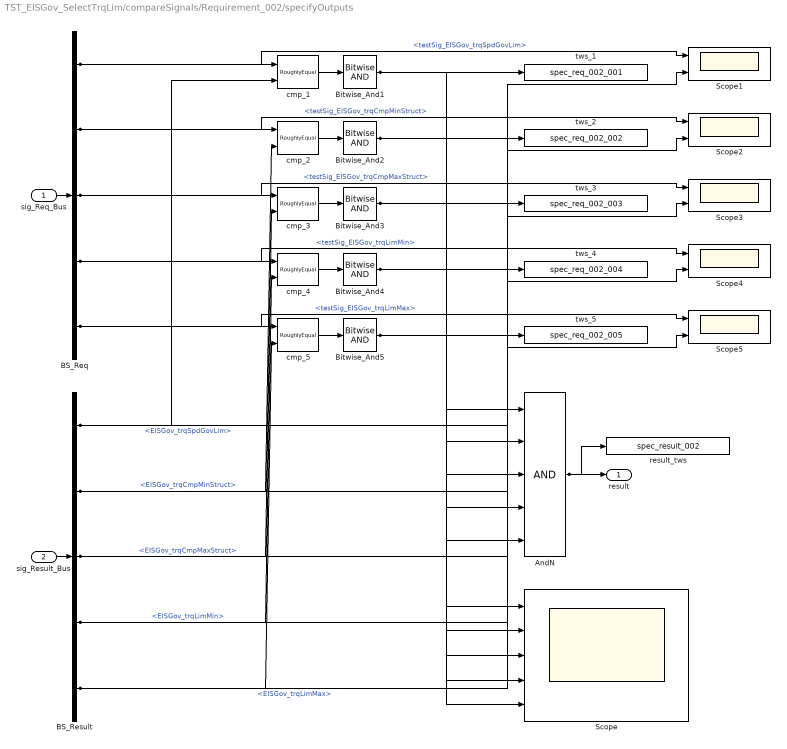
== system TST_EISGov_SelectTrqLim/compareSignals/Requirement_002/specifyOutputs ==
  sig_Req_Bus : Inport
  sig_Result_Bus : Inport  Port=2
  AndN : Logic  Inputs=5
  BS_Req : BusSelector  OutputSignals=testSig_EISGov_trqSpdGovLim,testSig_EISGov_trqCmpMinStruct,testSig_EISGov_trqCmpMaxStruct,testSig_EISGov_trqLimMin,testSig_EISGov_trqLimMax
  BS_Result : BusSelector  OutputSignals=EISGov_trqSpdGovLim,EISGov_trqCmpMinStruct,EISGov_trqCmpMaxStruct,EISGov_trqLimMin,EISGov_trqLimMax
  Bitwise_And{1..5} (5 alike) : simulink/Logic and Bit Operations/Bitwise Operator  logicop=AND  UseBitMask=off  BitMask=bin2dec('11011001')  BitMaskRealWorld=Stored Integer
  Scope : Scope  NumInputPorts=5
  Scope{1..5} (5 alike) : Scope  NumInputPorts=2
  cmp_{1..5} (5 alike) : UnitTest_Lib/RoughlyEqual  slope=0.1
  result_tws : ToWorkspace  VariableName=spec_result_002
  tws_1 : ToWorkspace  VariableName=spec_req_002_001
  tws_2 : ToWorkspace  VariableName=spec_req_002_002
  tws_3 : ToWorkspace  VariableName=spec_req_002_003
  tws_4 : ToWorkspace  VariableName=spec_req_002_004
  tws_5 : ToWorkspace  VariableName=spec_req_002_005
  result : Outport
  wires:
  sig_Req_Bus/1 -> BS_Req/1
  sig_Result_Bus/1 -> BS_Result/1
  AndN/1 -> result/1, result_tws/1
  BS_Req/1 -> cmp_1/1, Scope1/1  "<testSig_EISGov_trqSpdGovLim>"
  BS_Result/1 -> cmp_1/2, Scope1/2  "<EISGov_trqSpdGovLim>"
  cmp_1/1 -> Bitwise_And1/1
  Bitwise_And1/1 -> tws_1/1, AndN/1, Scope/1
  BS_Req/2 -> cmp_2/1, Scope2/1  "<testSig_EISGov_trqCmpMinStruct>"
  BS_Result/2 -> cmp_2/2, Scope2/2  "<EISGov_trqCmpMinStruct>"
  cmp_2/1 -> Bitwise_And2/1
  Bitwise_And2/1 -> tws_2/1, AndN/2, Scope/2
  BS_Req/3 -> cmp_3/1, Scope3/1  "<testSig_EISGov_trqCmpMaxStruct>"
  BS_Result/3 -> cmp_3/2, Scope3/2  "<EISGov_trqCmpMaxStruct>"
  cmp_3/1 -> Bitwise_And3/1
  Bitwise_And3/1 -> tws_3/1, AndN/3, Scope/3
  BS_Req/4 -> cmp_4/1, Scope4/1  "<testSig_EISGov_trqLimMin>"
  BS_Result/4 -> cmp_4/2, Scope4/2  "<EISGov_trqLimMin>"
  cmp_4/1 -> Bitwise_And4/1
  Bitwise_And4/1 -> tws_4/1, AndN/4, Scope/4
  BS_Req/5 -> cmp_5/1, Scope5/1  "<testSig_EISGov_trqLimMax>"
  BS_Result/5 -> cmp_5/2, Scope5/2  "<EISGov_trqLimMax>"
  cmp_5/1 -> Bitwise_And5/1
  Bitwise_And5/1 -> tws_5/1, AndN/5, Scope/5

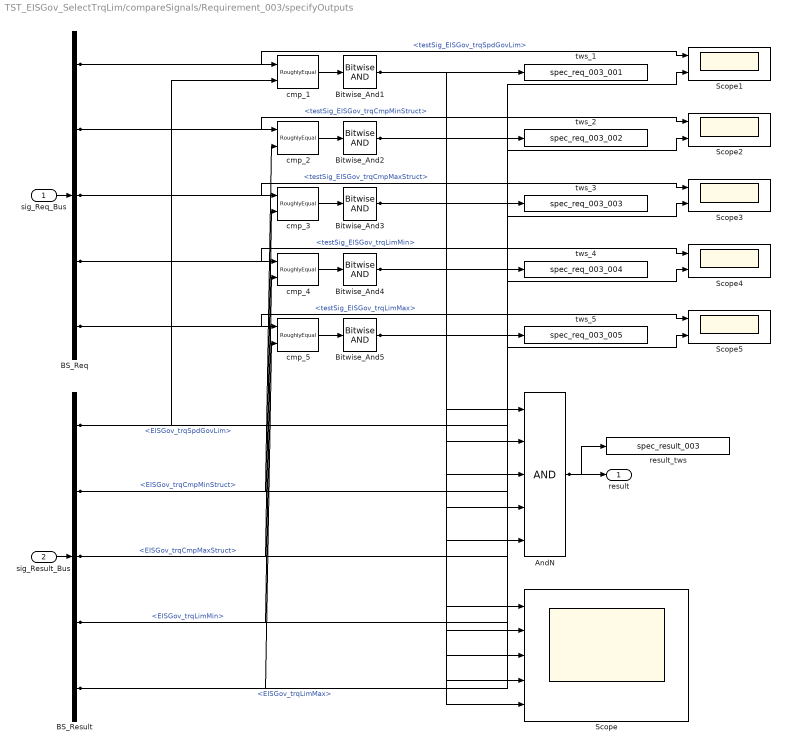
== system TST_EISGov_SelectTrqLim/compareSignals/Requirement_003/specifyOutputs ==
  sig_Req_Bus : Inport
  sig_Result_Bus : Inport  Port=2
  AndN : Logic  Inputs=5
  BS_Req : BusSelector  OutputSignals=testSig_EISGov_trqSpdGovLim,testSig_EISGov_trqCmpMinStruct,testSig_EISGov_trqCmpMaxStruct,testSig_EISGov_trqLimMin,testSig_EISGov_trqLimMax
  BS_Result : BusSelector  OutputSignals=EISGov_trqSpdGovLim,EISGov_trqCmpMinStruct,EISGov_trqCmpMaxStruct,EISGov_trqLimMin,EISGov_trqLimMax
  Bitwise_And{1..5} (5 alike) : simulink/Logic and Bit Operations/Bitwise Operator  logicop=AND  UseBitMask=off  BitMask=bin2dec('11011001')  BitMaskRealWorld=Stored Integer
  Scope : Scope  NumInputPorts=5
  Scope{1..5} (5 alike) : Scope  NumInputPorts=2
  cmp_{1..5} (5 alike) : UnitTest_Lib/RoughlyEqual  slope=0.1
  result_tws : ToWorkspace  VariableName=spec_result_003
  tws_1 : ToWorkspace  VariableName=spec_req_003_001
  tws_2 : ToWorkspace  VariableName=spec_req_003_002
  tws_3 : ToWorkspace  VariableName=spec_req_003_003
  tws_4 : ToWorkspace  VariableName=spec_req_003_004
  tws_5 : ToWorkspace  VariableName=spec_req_003_005
  result : Outport
  wires:
  sig_Req_Bus/1 -> BS_Req/1
  sig_Result_Bus/1 -> BS_Result/1
  AndN/1 -> result/1, result_tws/1
  BS_Req/1 -> cmp_1/1, Scope1/1  "<testSig_EISGov_trqSpdGovLim>"
  BS_Result/1 -> cmp_1/2, Scope1/2  "<EISGov_trqSpdGovLim>"
  cmp_1/1 -> Bitwise_And1/1
  Bitwise_And1/1 -> tws_1/1, AndN/1, Scope/1
  BS_Req/2 -> cmp_2/1, Scope2/1  "<testSig_EISGov_trqCmpMinStruct>"
  BS_Result/2 -> cmp_2/2, Scope2/2  "<EISGov_trqCmpMinStruct>"
  cmp_2/1 -> Bitwise_And2/1
  Bitwise_And2/1 -> tws_2/1, AndN/2, Scope/2
  BS_Req/3 -> cmp_3/1, Scope3/1  "<testSig_EISGov_trqCmpMaxStruct>"
  BS_Result/3 -> cmp_3/2, Scope3/2  "<EISGov_trqCmpMaxStruct>"
  cmp_3/1 -> Bitwise_And3/1
  Bitwise_And3/1 -> tws_3/1, AndN/3, Scope/3
  BS_Req/4 -> cmp_4/1, Scope4/1  "<testSig_EISGov_trqLimMin>"
  BS_Result/4 -> cmp_4/2, Scope4/2  "<EISGov_trqLimMin>"
  cmp_4/1 -> Bitwise_And4/1
  Bitwise_And4/1 -> tws_4/1, AndN/4, Scope/4
  BS_Req/5 -> cmp_5/1, Scope5/1  "<testSig_EISGov_trqLimMax>"
  BS_Result/5 -> cmp_5/2, Scope5/2  "<EISGov_trqLimMax>"
  cmp_5/1 -> Bitwise_And5/1
  Bitwise_And5/1 -> tws_5/1, AndN/5, Scope/5
